simulink model "ControlComparison"  (R2018a)
settings: Solver=VariableStepAuto  StartTime=0  StopTime=4  FixedStep=1e-6
undefined symbols (not defined in the file): alternator, electrical_load, i_f_max, iceToAltRotRatio, n_ice_f, n_ice_i, normalizationFactor, rectifier, t_brake_f, t_brake_i, T_k, T_s
libraries: elec_lib x36, fl_lib x29, nesl_utility x26, neural x25, simulink x6, SimscapeCustomBlocks_lib x2
(part 1 of 3)
settings Model: Creator=gabrielrodrigues  LastModifiedBy=gabriel.rodrigues
settings DataIOCC: ReturnWorkspaceOutputs=on
settings CodeAppCC: StateflowObjectComments=on
settings SimscapeCC: SimscapeNormalizeSystem=off  SimscapeLogType=local  SimscapeLogLimitData=off

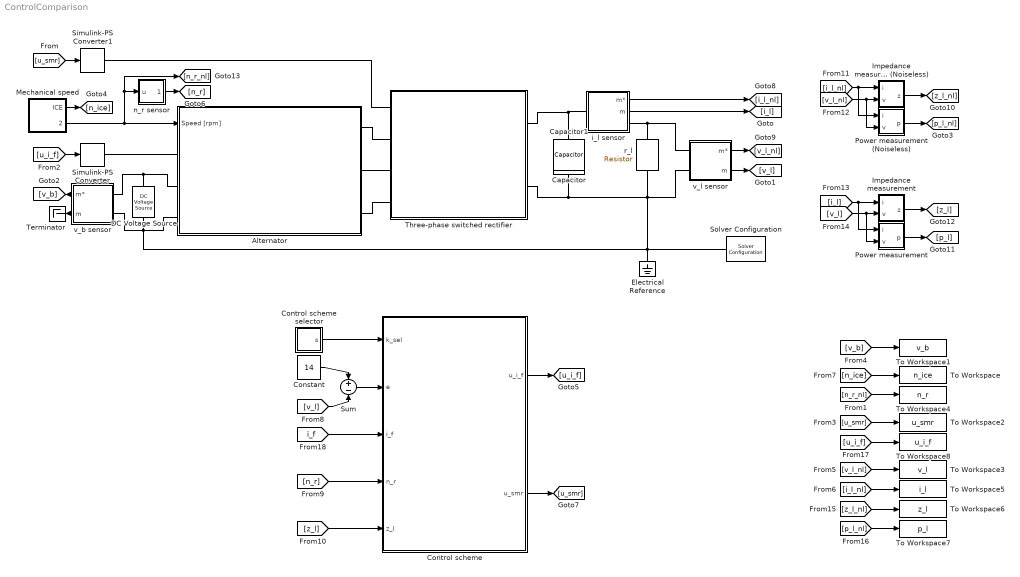
== system ControlComparison ==
  Alternator : Subsystem
  Capacitor : fl_lib/Electrical/Electrical Elements/Capacitor  c=10e-3 F  r=1e-6 Ohm  g=0 1/Ohm  i_specify=off  i_priority=None  i=0 A  i_nominal_specify=off  i_nominal_unit=A  i_nominal_value=1  v_specify=off  v_priority=None  v=0 V  v_nominal_specify=off  v_nominal_unit=V  v_nominal_value=1  vc_specify=off  vc_priority=High  vc=0 V  vc_nominal_specify=off  vc_nominal_unit=V  vc_nominal_value=1
  Capacitor1 : fl_lib/Electrical/Electrical Elements/Capacitor  c=rectifier.filter.c F  r=1e-6 Ohm  g=0 1/Ohm  i_specify=off  i_priority=None  i=0 A  i_nominal_specify=off  i_nominal_unit=A  i_nominal_value=1  v_specify=off  v_priority=None  v=0 V  v_nominal_specify=off  v_nominal_unit=V  v_nominal_value=1  vc_specify=off  vc_priority=High  vc=0 V  vc_nominal_specify=off  vc_nominal_unit=V  vc_nominal_value=1
  Constant : Constant  Value=14
  Control scheme : Subsystem  Variant=on
  Control scheme selector : Subsystem  mask{s_i=0, s_f=1, t_i=t_brake_i, t_f=t_brake_f}
      mask prompts: s_i "Initial value"; s_f "Final value"; t_i "Step start [s]"; t_f "Step end [s]"
  DC Voltage Source : elec_lib/Additional Components/SPICE-Compatible Components/Sources/DC Voltage Source  DC=alternator.rotor.r.value * i_f_max V
      settings: SourceProductName=Simscape Electronics  SourceProductBaseCode=SN
  Electrical Reference : fl_lib/Electrical/Electrical Elements/Electrical Reference
  Impedance measurement : Subsystem
  Impedance measurement (Noiseless) : Subsystem
  Mechanical speed : Subsystem
  Power measurement : Subsystem
  Power measurement (Noiseless) : Subsystem
  Simulink-PS Converter : nesl_utility/Simulink-PS Converter  PhysicalDomain=network_engine_domain  SubClassName=ps_input  LeftPortType=input  RightPortType=output  PseudoPeriodic=off  Frequencies=[]  NoiseDistribution=none  NoiseParameters=[]  Unit=1  AffineConversion=off  FilteringAndDerivatives=provide  SimscapeFilterOrder=1  InputFilterTimeConstant=0.001  UdotUserProvided=0
  Simulink-PS Converter1 : nesl_utility/Simulink-PS Converter  PhysicalDomain=network_engine_domain  SubClassName=ps_input  LeftPortType=input  RightPortType=output  PseudoPeriodic=off  Frequencies=[]  NoiseDistribution=none  NoiseParameters=[]  Unit=1  AffineConversion=off  FilteringAndDerivatives=provide  SimscapeFilterOrder=1  InputFilterTimeConstant=0.001  UdotUserProvided=0
  Solver Configuration : nesl_utility/Solver Configuration  PhysicalDomain=network_engine_domain  SubClassName=solver  LeftPortType=input  RightPortType=generic  Tones=[]  Harmonics=[]  SimulateNoise=off  Profile=off  UseLocalSampling=off  EnableSwitchedLinearOptims=on  FrequencyDomain=off  UseCCode=off  RelTol=0.001  AbsTol=1e-06  MinStep=1e-09  ToWorkspace=off  RevertToSquareIcSolve=off  NumHomotopyIterations=100  PhasorMode=off  PhasorModeNumHarmonics=1  DoDC=on  ResidualTolerance=1e-09  UseLocalSolver=on  LocalSolverChoice=NE_TRAPEZOIDAL_ADVANCER  LocalSolverSampleTime=1e-06  DoFixedCost=on  MaxNonlinIter=20  MaxModeIter=2  LinearAlgebra=Sparse  EquationFormulation=NE_TIME_EF  DelaysMemoryBudget=1024  AutomaticFiltering=on  FilteringTimeConstant=0.001  PartitionStorageMethod=AS_NEEDED  PartitionMemoryBudget=1024
  Sum : Sum  Inputs=+-
  Terminator : Terminator
  Three-phase switched rectifier : Subsystem
  To Workspace : ToWorkspace  VariableName=n_ice  SaveFormat=Timeseries  SampleTime=-1
  To Workspace1 : ToWorkspace  VariableName=v_b  SaveFormat=Timeseries  SampleTime=-1
  To Workspace2 : ToWorkspace  VariableName=u_smr  SaveFormat=Timeseries  SampleTime=-1
  To Workspace3 : ToWorkspace  VariableName=v_l  SaveFormat=Timeseries  SampleTime=-1
  To Workspace4 : ToWorkspace  VariableName=n_r  SaveFormat=Timeseries  SampleTime=-1
  To Workspace5 : ToWorkspace  VariableName=i_l  SaveFormat=Timeseries  SampleTime=-1
  To Workspace6 : ToWorkspace  VariableName=z_l  SaveFormat=Timeseries  SampleTime=-1
  To Workspace7 : ToWorkspace  VariableName=p_l  SaveFormat=Timeseries  SampleTime=-1
  To Workspace8 : ToWorkspace  VariableName=u_i_f  SaveFormat=Timeseries  SampleTime=-1
  i_l sensor : Subsystem
  n_r sensor : Subsystem  mask{T_s=T_s, seed=1515, noise=0.001}
      mask prompts: T_s "Sample time [s]"; noise "Noise percentage"
      mask DialogControl DescGroupVar Prompt: Noisy voltage sensor
  r_l : elec_lib/Passive Devices/Resistor  R=electrical_load.r Ohm  R_tol=5  enable_R_tol=0  tol_distribution=1  nSigma=4  enable_operating_limits=0  operating_limit_action=2  max_working_voltage=100 V  power_rating=1 W  enable_faults=0  fault_action=1  R_faulted=inf Ohm  enable_temporal_fault=0  t_fault=1 s  enable_behavioral_fault=0  max_permissible_current=1 A  t_fail_on_current=1 s  noise_mode=0  sample_time=1e-3 s  repeatability=1  auto_seed=3922919431  user_seed=0  Tdevice=25 degC  alpha=3.93e-3 1/K  Tmeas=25 degC  thermal_mass=100 J/K  power_derating_T1=70 degC  power_derating_T2=155 degC  operating_temperature_range_vec=[-50, 150] degC  temperature_specify=off  temperature_priority=High  temperature=298.15 K  temperature_nominal_specify=off  temperature_nominal_unit=K  temperature_nominal_value=1
  v_b sensor : Subsystem
  v_l sensor : Subsystem
  wires:
  Mechanical speed/2(Alternator) -> [n_r_nl], n_r sensor/1(u), Alternator/1(Speed [rpm])
  [u_i_f] -> Simulink-PS Converter/1
  [u_smr] -> Simulink-PS Converter1/1
  Constant/1 -> Sum/1
  [u_smr] -> To Workspace2/1
  [v_b] -> To Workspace1/1
  [i_l_nl] -> To Workspace5/1
  [v_l_nl] -> To Workspace3/1
  Mechanical speed/1(ICE) -> [n_ice]
  [n_r_nl] -> To Workspace4/1
  [n_ice] -> To Workspace/1
  [v_l] -> Sum/2
  n_r sensor/1(m) -> [n_r]
  v_l sensor/2(m) -> [v_l]
  i_l sensor/2(m) -> [i_l]
  i_l sensor/1(m*) -> [i_l_nl]
  v_l sensor/1(m*) -> [v_l_nl]
  Power measurement (Noiseless)/1(p) -> [p_l_nl]
  Impedance measurement (Noiseless)/1(z) -> [z_l_nl]
  Power measurement/1(p) -> [p_l]
  Impedance measurement/1(z) -> [z_l]
  v_b sensor/1(m*) -> [v_b]
  v_b sensor/2(m) -> Terminator/1
  [i_l_nl] -> Power measurement (Noiseless)/1(i), Impedance measurement (Noiseless)/1(i)
  [v_l_nl] -> Power measurement (Noiseless)/2(v), Impedance measurement (Noiseless)/2(v)
  [v_l] -> Impedance measurement/2(v), Power measurement/2(v)
  [i_l] -> Impedance measurement/1(i), Power measurement/1(i)
  Control scheme/1(u_i_f) -> [u_i_f]
  Control scheme/2(u_smr) -> [u_smr]
  Control scheme selector/1(s) -> Control scheme/1(k_sel)
  [z_l] -> Control scheme/5(z_l)
  [n_r] -> Control scheme/4(n_r)
  Sum/1 -> Control scheme/2(e)
  [p_l_nl] -> To Workspace7/1
  [z_l_nl] -> To Workspace6/1
  [u_i_f] -> To Workspace8/1
  [i_f] -> Control scheme/3(i_f)
  connections:
  Three-phase switched rectifier/LConn3 -- Alternator/RConn2
  Three-phase switched rectifier/LConn4 -- Alternator/RConn3
  Three-phase switched rectifier/LConn2 -- Alternator/RConn1
  Solver Configuration/RConn1 -- Electrical Reference/LConn1 -- v_b sensor/LConn2 -- DC Voltage Source/RConn1 -- Alternator/LConn3 -- r_l/RConn1 -- v_l sensor/LConn2 -- Capacitor/RConn1 -- Three-phase switched rectifier/RConn2
  i_l sensor/RConn1 -- v_l sensor/LConn1 -- r_l/LConn1
  Capacitor/LConn1 -- i_l sensor/LConn1 -- Three-phase switched rectifier/RConn1
  Alternator/LConn2 -- v_b sensor/LConn1 -- DC Voltage Source/LConn1
  Three-phase switched rectifier/LConn1 -- Simulink-PS Converter1/RConn1
  Simulink-PS Converter/RConn1 -- Alternator/LConn1

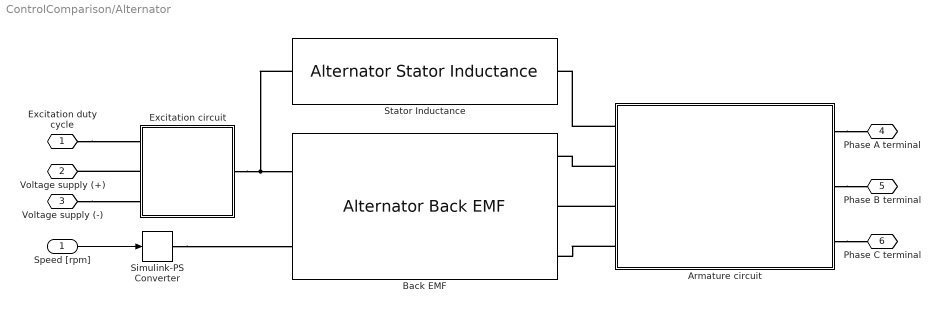
== system ControlComparison/Alternator ==
  Speed [rpm] : Inport
  Armature circuit : Subsystem  Variant=on
  Back EMF : SimscapeCustomBlocks_lib/Alternator/Alternator Back EMF  p=alternator.p  omega_r_specify=off  omega_r_priority=None  omega_r=0 rad/s  omega_r_nominal_specify=off  omega_r_nominal_unit=rad/s  omega_r_nominal_value=1  omega_e_specify=off  omega_e_priority=None  omega_e=0 rad/s  omega_e_nominal_specify=off  omega_e_nominal_unit=rad/s  omega_e_nominal_value=1  k_e_specify=off  k_e_priority=None  k_e=0 s*V/rad/A  k_e_nominal_specify=off  k_e_nominal_unit=s*V/rad/A  k_e_nominal_value=1  e_specify=off  e_priority=None  e=0 rpm  e_nominal_specify=off  e_nominal_unit=rpm  e_nominal_value=1
  Excitation circuit : Subsystem
  Simulink-PS Converter : nesl_utility/Simulink-PS Converter  PhysicalDomain=network_engine_domain  SubClassName=ps_input  LeftPortType=input  RightPortType=output  PseudoPeriodic=off  Frequencies=[]  NoiseDistribution=none  NoiseParameters=[]  Unit=1  AffineConversion=off  FilteringAndDerivatives=provide  SimscapeFilterOrder=1  InputFilterTimeConstant=0.001  UdotUserProvided=0
  Stator Inductance : SimscapeCustomBlocks_lib/Alternator/Alternator Stator Inductance
  Excitation duty cycle : PMIOPort  Side=Left
  Voltage supply (+) : PMIOPort  Port=2  Side=Left
  Voltage supply (-) : PMIOPort  Port=3  Side=Left
  Phase A terminal : PMIOPort  Port=4  Side=Right
  Phase B terminal : PMIOPort  Port=5  Side=Right
  Phase C terminal : PMIOPort  Port=6  Side=Right
  wires:
  Speed [rpm]/1 -> Simulink-PS Converter/1
  connections:
  Armature circuit/RConn1 -- Phase A terminal/RConn1
  Armature circuit/RConn2 -- Phase B terminal/RConn1
  Excitation circuit/LConn2 -- Voltage supply (+)/RConn1
  Voltage supply (-)/RConn1 -- Excitation circuit/LConn3
  Armature circuit/LConn3 -- Back EMF/RConn2
  Armature circuit/LConn2 -- Back EMF/RConn1
  Armature circuit/LConn4 -- Back EMF/RConn3
  Simulink-PS Converter/RConn1 -- Back EMF/LConn2
  Armature circuit/LConn1 -- Stator Inductance/RConn1
  Excitation duty cycle/RConn1 -- Excitation circuit/LConn1
  Excitation circuit/RConn1 -- Stator Inductance/LConn1 -- Back EMF/LConn1
  Armature circuit/RConn3 -- Phase C terminal/RConn1

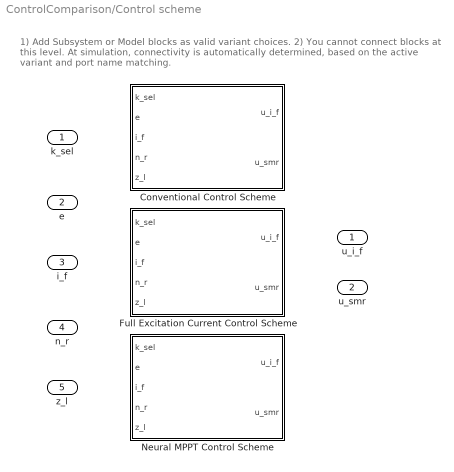
== system ControlComparison/Control scheme ==
  note: 1) Add Subsystem or Model blocks as valid variant choices.
      | 2) You cannot connect blocks at this level. At simulation, connectivity is automatically
      | determined, based on the active variant and port name matching.
  k_sel : Inport
  e : Inport  Port=2
  i_f : Inport  Port=3
  n_r : Inport  Port=4
  z_l : Inport  Port=5
  Conventional Control Scheme : Subsystem  VariantControl=conventionalControlScheme
  Full Excitation Current Control Scheme : Subsystem  VariantControl=fullExcitationCurrentControlScheme
  Neural MPPT Control Scheme : Subsystem  VariantControl=neuralControlScheme
  u_i_f : Outport
  u_smr : Outport  Port=2

== system ControlComparison/Control scheme selector ==
  Step off : Step  Time=t_f  After=s_f - s_i  SampleTime=0
  Step on : Step  Time=t_i  Before=s_i  After=s_f  SampleTime=0
  Sum : Sum  Inputs=+-
  s : Outport
  wires:
  Sum/1 -> s/1
  Step off/1 -> Sum/2
  Step on/1 -> Sum/1

== system ControlComparison/Impedance measurement ==
  i : Inport
  v : Inport  Port=2
  MATLAB Function : MATLAB Function  TreatAsAtomicUnit=on
  z : Outport
  wires:
  i/1 -> MATLAB Function/2(i)
  v/1 -> MATLAB Function/1(v)
  MATLAB Function/1(z) -> z/1

== system ControlComparison/Impedance measurement (Noiseless) ==
  i : Inport
  v : Inport  Port=2
  MATLAB Function : MATLAB Function  TreatAsAtomicUnit=on
  z : Outport
  wires:
  MATLAB Function/1(z) -> z/1
  v/1 -> MATLAB Function/1(v)
  i/1 -> MATLAB Function/2(i)

== system ControlComparison/Mechanical speed ==
  ICE Speed : Subsystem  mask{s_i=n_ice_i, s_f=n_ice_f, t_i=t_brake_i, t_f=t_brake_f}
      mask prompts: s_i "Initial value"; s_f "Final value"; t_i "Ramp start [s]"; t_f "Ramp end [s]"
  ICE to Alternator Rotation Ratio : Constant  Value=iceToAltRotRatio
  Product : Product
  ICE : Outport
  Alternator : Outport  Port=2
  wires:
  ICE Speed/1(s) -> ICE/1, Product/1
  ICE to Alternator Rotation Ratio/1 -> Product/2
  Product/1 -> Alternator/1

== system ControlComparison/Power measurement ==
  i : Inport
  v : Inport  Port=2
  Product : Product
  p : Outport
  wires:
  i/1 -> Product/2
  v/1 -> Product/1
  Product/1 -> p/1

== system ControlComparison/Power measurement (Noiseless) ==
  i : Inport
  v : Inport  Port=2
  Product : Product
  p : Outport
  wires:
  i/1 -> Product/2
  v/1 -> Product/1
  Product/1 -> p/1

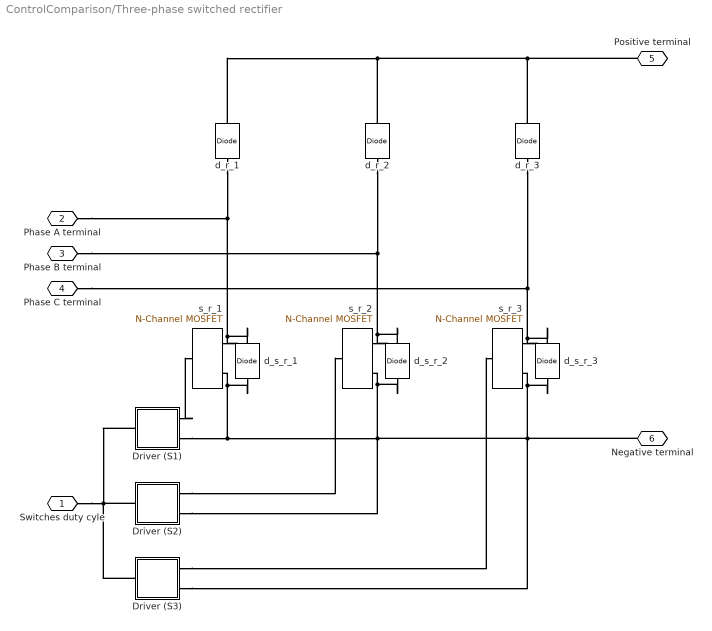
== system ControlComparison/Three-phase switched rectifier ==
  Driver (S1) : Subsystem
  Driver (S2) : Subsystem
  Driver (S3) : Subsystem
  d_r_1 : elec_lib/Semiconductor Devices/Diode  ModelType=1  Vf=rectifier.d.v_on V  Ron=rectifier.d.r_on Ohm  Goff=1e-8 S  Rz=0.3 Ohm  Vz=50 V  C_PWL=5 pF  prmExp=1  I12=[.0137, .545] A  V12=[.6, .7] V  I1=0.0137 A  V1=0.6 V  IS=1e-12 A  ec=1  RS=0.01 Ohm  Tmeas=25 degC  BV=inf V  C_param=1  CJ0=5 pF  VJ=1 V  Mgrad=0.5  Vvec=[.1, 10, 100] V  Cvec=[3.5, 1, .4] pF  FC=0.5  Q_param=1  Irrm=-7.15 A  iF=4 A  didt=-750 A/us  trr=115 ns  TT=50 ns  tau=100 ns  T_param=1  IS_T2=1.25e-7 A  I1_T2=0.245 A  V1_T2=0.5 V  Tmeas2=125 degC  EG_param=1  EG=1.11 eV  XTI_param=1  XTI=3  dBVdT=0 V/K  Tdevice=25 degC  i_capacitor_specify=off  i_capacitor_priority=High  i_capacitor=0 A  i_capacitor_nominal_specify=off  i_capacitor_nominal_unit=A  i_capacitor_nominal_value=1  v_capacitor_specify=off  v_capacitor_priority=None  v_capacitor=0 V  v_capacitor_nominal_specify=off  v_capacitor_nominal_unit=V  v_capacitor_nominal_value=1  Rth=[0, 10] K/W  thermal_mass_parameterization=1  thermal_mass=[0, 1] J/K  thermal_time_constant=[0, 10] s  thermal_mass_initial_temperatures=[25, 25] degC
      settings: SourceProductName=Simscape Electronics  SourceProductBaseCode=SN
  d_r_2 : elec_lib/Semiconductor Devices/Diode  ModelType=1  Vf=rectifier.d.v_on V  Ron=rectifier.d.r_on Ohm  Goff=1e-8 S  Rz=0.3 Ohm  Vz=50 V  C_PWL=5 pF  prmExp=1  I12=[.0137, .545] A  V12=[.6, .7] V  I1=0.0137 A  V1=0.6 V  IS=1e-12 A  ec=1  RS=0.01 Ohm  Tmeas=25 degC  BV=inf V  C_param=1  CJ0=5 pF  VJ=1 V  Mgrad=0.5  Vvec=[.1, 10, 100] V  Cvec=[3.5, 1, .4] pF  FC=0.5  Q_param=1  Irrm=-7.15 A  iF=4 A  didt=-750 A/us  trr=115 ns  TT=50 ns  tau=100 ns  T_param=1  IS_T2=1.25e-7 A  I1_T2=0.245 A  V1_T2=0.5 V  Tmeas2=125 degC  EG_param=1  EG=1.11 eV  XTI_param=1  XTI=3  dBVdT=0 V/K  Tdevice=25 degC  i_capacitor_specify=off  i_capacitor_priority=High  i_capacitor=0 A  i_capacitor_nominal_specify=off  i_capacitor_nominal_unit=A  i_capacitor_nominal_value=1  v_capacitor_specify=off  v_capacitor_priority=None  v_capacitor=0 V  v_capacitor_nominal_specify=off  v_capacitor_nominal_unit=V  v_capacitor_nominal_value=1  Rth=[0, 10] K/W  thermal_mass_parameterization=1  thermal_mass=[0, 1] J/K  thermal_time_constant=[0, 10] s  thermal_mass_initial_temperatures=[25, 25] degC
      settings: SourceProductName=Simscape Electronics  SourceProductBaseCode=SN
  d_r_3 : elec_lib/Semiconductor Devices/Diode  ModelType=1  Vf=rectifier.d.v_on V  Ron=rectifier.d.r_on Ohm  Goff=1e-8 S  Rz=0.3 Ohm  Vz=50 V  C_PWL=5 pF  prmExp=1  I12=[.0137, .545] A  V12=[.6, .7] V  I1=0.0137 A  V1=0.6 V  IS=1e-12 A  ec=1  RS=0.01 Ohm  Tmeas=25 degC  BV=inf V  C_param=1  CJ0=5 pF  VJ=1 V  Mgrad=0.5  Vvec=[.1, 10, 100] V  Cvec=[3.5, 1, .4] pF  FC=0.5  Q_param=1  Irrm=-7.15 A  iF=4 A  didt=-750 A/us  trr=115 ns  TT=50 ns  tau=100 ns  T_param=1  IS_T2=1.25e-7 A  I1_T2=0.245 A  V1_T2=0.5 V  Tmeas2=125 degC  EG_param=1  EG=1.11 eV  XTI_param=1  XTI=3  dBVdT=0 V/K  Tdevice=25 degC  i_capacitor_specify=off  i_capacitor_priority=High  i_capacitor=0 A  i_capacitor_nominal_specify=off  i_capacitor_nominal_unit=A  i_capacitor_nominal_value=1  v_capacitor_specify=off  v_capacitor_priority=None  v_capacitor=0 V  v_capacitor_nominal_specify=off  v_capacitor_nominal_unit=V  v_capacitor_nominal_value=1  Rth=[0, 10] K/W  thermal_mass_parameterization=1  thermal_mass=[0, 1] J/K  thermal_time_constant=[0, 10] s  thermal_mass_initial_temperatures=[25, 25] degC
      settings: SourceProductName=Simscape Electronics  SourceProductBaseCode=SN
  d_s_r_1 : elec_lib/Semiconductor Devices/Diode  ModelType=1  Vf=rectifier.d.v_on V  Ron=rectifier.d.r_on Ohm  Goff=1e-8 S  Rz=0.3 Ohm  Vz=50 V  C_PWL=5 pF  prmExp=1  I12=[.0137, .545] A  V12=[.6, .7] V  I1=0.0137 A  V1=0.6 V  IS=1e-12 A  ec=1  RS=0.01 Ohm  Tmeas=25 degC  BV=inf V  C_param=1  CJ0=5 pF  VJ=1 V  Mgrad=0.5  Vvec=[.1, 10, 100] V  Cvec=[3.5, 1, .4] pF  FC=0.5  Q_param=1  Irrm=-7.15 A  iF=4 A  didt=-750 A/us  trr=115 ns  TT=50 ns  tau=100 ns  T_param=1  IS_T2=1.25e-7 A  I1_T2=0.245 A  V1_T2=0.5 V  Tmeas2=125 degC  EG_param=1  EG=1.11 eV  XTI_param=1  XTI=3  dBVdT=0 V/K  Tdevice=25 degC  i_capacitor_specify=off  i_capacitor_priority=High  i_capacitor=0 A  i_capacitor_nominal_specify=off  i_capacitor_nominal_unit=A  i_capacitor_nominal_value=1  v_capacitor_specify=off  v_capacitor_priority=None  v_capacitor=0 V  v_capacitor_nominal_specify=off  v_capacitor_nominal_unit=V  v_capacitor_nominal_value=1  Rth=[0, 10] K/W  thermal_mass_parameterization=1  thermal_mass=[0, 1] J/K  thermal_time_constant=[0, 10] s  thermal_mass_initial_temperatures=[25, 25] degC
      settings: SourceProductName=Simscape Electronics  SourceProductBaseCode=SN
  d_s_r_2 : elec_lib/Semiconductor Devices/Diode  ModelType=1  Vf=rectifier.d.v_on V  Ron=rectifier.d.r_on Ohm  Goff=1e-8 S  Rz=0.3 Ohm  Vz=50 V  C_PWL=5 pF  prmExp=1  I12=[.0137, .545] A  V12=[.6, .7] V  I1=0.0137 A  V1=0.6 V  IS=1e-12 A  ec=1  RS=0.01 Ohm  Tmeas=25 degC  BV=inf V  C_param=1  CJ0=5 pF  VJ=1 V  Mgrad=0.5  Vvec=[.1, 10, 100] V  Cvec=[3.5, 1, .4] pF  FC=0.5  Q_param=1  Irrm=-7.15 A  iF=4 A  didt=-750 A/us  trr=115 ns  TT=50 ns  tau=100 ns  T_param=1  IS_T2=1.25e-7 A  I1_T2=0.245 A  V1_T2=0.5 V  Tmeas2=125 degC  EG_param=1  EG=1.11 eV  XTI_param=1  XTI=3  dBVdT=0 V/K  Tdevice=25 degC  i_capacitor_specify=off  i_capacitor_priority=High  i_capacitor=0 A  i_capacitor_nominal_specify=off  i_capacitor_nominal_unit=A  i_capacitor_nominal_value=1  v_capacitor_specify=off  v_capacitor_priority=None  v_capacitor=0 V  v_capacitor_nominal_specify=off  v_capacitor_nominal_unit=V  v_capacitor_nominal_value=1  Rth=[0, 10] K/W  thermal_mass_parameterization=1  thermal_mass=[0, 1] J/K  thermal_time_constant=[0, 10] s  thermal_mass_initial_temperatures=[25, 25] degC
      settings: SourceProductName=Simscape Electronics  SourceProductBaseCode=SN
  d_s_r_3 : elec_lib/Semiconductor Devices/Diode  ModelType=1  Vf=rectifier.d.v_on V  Ron=rectifier.d.r_on Ohm  Goff=1e-8 S  Rz=0.3 Ohm  Vz=50 V  C_PWL=5 pF  prmExp=1  I12=[.0137, .545] A  V12=[.6, .7] V  I1=0.0137 A  V1=0.6 V  IS=1e-12 A  ec=1  RS=0.01 Ohm  Tmeas=25 degC  BV=inf V  C_param=1  CJ0=5 pF  VJ=1 V  Mgrad=0.5  Vvec=[.1, 10, 100] V  Cvec=[3.5, 1, .4] pF  FC=0.5  Q_param=1  Irrm=-7.15 A  iF=4 A  didt=-750 A/us  trr=115 ns  TT=50 ns  tau=100 ns  T_param=1  IS_T2=1.25e-7 A  I1_T2=0.245 A  V1_T2=0.5 V  Tmeas2=125 degC  EG_param=1  EG=1.11 eV  XTI_param=1  XTI=3  dBVdT=0 V/K  Tdevice=25 degC  i_capacitor_specify=off  i_capacitor_priority=High  i_capacitor=0 A  i_capacitor_nominal_specify=off  i_capacitor_nominal_unit=A  i_capacitor_nominal_value=1  v_capacitor_specify=off  v_capacitor_priority=None  v_capacitor=0 V  v_capacitor_nominal_specify=off  v_capacitor_nominal_unit=V  v_capacitor_nominal_value=1  Rth=[0, 10] K/W  thermal_mass_parameterization=1  thermal_mass=[0, 1] J/K  thermal_time_constant=[0, 10] s  thermal_mass_initial_temperatures=[25, 25] degC
      settings: SourceProductName=Simscape Electronics  SourceProductBaseCode=SN
  s_r_1 : elec_lib/Semiconductor Devices/N-Channel MOSFET  parameterization=1  prmDatasheet=1  prmEquCoeff=1  Beta=5 A/V^2  Rds=0.025 Ohm  Id=6 A  Vgs=rectifier.s.v_gs_on V  Vth=1.7 V  lam=0 1/V  Tmeas=25 degC  RS=1e-4 Ohm  RD=0.01 Ohm  C_param=1  C_GS=270 pF  C_GD=80 pF  C_DS=0 pF  C_iss=350 pF  C_rss=80 pF  C_oss=0 pF  C_GS_vec=[ 270 300 290 280 295 255 ] pF  C_GD_vec=[ 450 400 300 190 95 55 ] pF  C_DS_vec=[ 450 410 390 230 175 115 ] pF  C_iss_vec=[ 720 700 590 470 390 310 ] pF  C_rss_vec=[ 450 400 300 190 95 55 ] pF  C_oss_vec=[ 900 810 690 420 270 170 ] pF  C_Vds_vec=[ 0.1 0.3 1 3 10 30 ] V  V_GS_for_cap_data=0 V  charge_linearity_param=1  C_OX=200 pF  V_C_OX=-0.5 V  IsDiode=0 A  Vbi=0.6 V  n=1  Cj0Diode=0 pF  TT=50e-9 s  dVth_dT=-6 mV/K  Rds_T2=0.037 Ohm  Tmeas2=125 degC  BEXDatasheet=-1.5  BEXEquCoeff=-1.5  etaisDatasheet=3  etaisEquCoeff=3  TdeviceDatasheet=25 degC  TdeviceEquCoeff=25 degC  Rth=[1, 10] K/W  thermal_mass_parameterization=1  thermal_mass=[1, 1] J/K  thermal_time_constant=[1, 10] s  thermal_mass_initial_temperatures=[ 25 25 ] degC  betaref=18 A/V^2  Vfbref=-1.1 V  gamma=3.5 V^0.50000  phib2ref=1 V  thesatref=0.4 1/V  alpha=0  Vp=5e-2 V  thesrref=0 1/V  m=8  Tref=25 degC  Cox=1500 pF  Cgso=100 pF  Cgdo=14 pF  Rsref=2e-3 Ohm  Rdref=0.17 Ohm  Rgref=8.4 Ohm  Isref=5.2e-13 A  Cj0=480 pF  Tprm=1  etabet=1.3  Stvfb=5e-4 V/K  Stphib=-8.5e-4 V/K  etasat=1.04  etasr=0.65  etar=0.95  etais=3  Tsim=25 degC  T0=[25, 25] degC
      settings: SourceProductName=Simscape Electronics  SourceProductBaseCode=SN  LogSimulationData=on
  s_r_2 : elec_lib/Semiconductor Devices/N-Channel MOSFET  parameterization=1  prmDatasheet=1  prmEquCoeff=1  Beta=5 A/V^2  Rds=0.025 Ohm  Id=6 A  Vgs=rectifier.s.v_gs_on V  Vth=1.7 V  lam=0 1/V  Tmeas=25 degC  RS=1e-4 Ohm  RD=0.01 Ohm  C_param=1  C_GS=270 pF  C_GD=80 pF  C_DS=0 pF  C_iss=350 pF  C_rss=80 pF  C_oss=0 pF  C_GS_vec=[ 270 300 290 280 295 255 ] pF  C_GD_vec=[ 450 400 300 190 95 55 ] pF  C_DS_vec=[ 450 410 390 230 175 115 ] pF  C_iss_vec=[ 720 700 590 470 390 310 ] pF  C_rss_vec=[ 450 400 300 190 95 55 ] pF  C_oss_vec=[ 900 810 690 420 270 170 ] pF  C_Vds_vec=[ 0.1 0.3 1 3 10 30 ] V  V_GS_for_cap_data=0 V  charge_linearity_param=1  C_OX=200 pF  V_C_OX=-0.5 V  IsDiode=0 A  Vbi=0.6 V  n=1  Cj0Diode=0 pF  TT=50e-9 s  dVth_dT=-6 mV/K  Rds_T2=0.037 Ohm  Tmeas2=125 degC  BEXDatasheet=-1.5  BEXEquCoeff=-1.5  etaisDatasheet=3  etaisEquCoeff=3  TdeviceDatasheet=25 degC  TdeviceEquCoeff=25 degC  Rth=[1, 10] K/W  thermal_mass_parameterization=1  thermal_mass=[1, 1] J/K  thermal_time_constant=[1, 10] s  thermal_mass_initial_temperatures=[ 25 25 ] degC  betaref=18 A/V^2  Vfbref=-1.1 V  gamma=3.5 V^0.50000  phib2ref=1 V  thesatref=0.4 1/V  alpha=0  Vp=5e-2 V  thesrref=0 1/V  m=8  Tref=25 degC  Cox=1500 pF  Cgso=100 pF  Cgdo=14 pF  Rsref=2e-3 Ohm  Rdref=0.17 Ohm  Rgref=8.4 Ohm  Isref=5.2e-13 A  Cj0=480 pF  Tprm=1  etabet=1.3  Stvfb=5e-4 V/K  Stphib=-8.5e-4 V/K  etasat=1.04  etasr=0.65  etar=0.95  etais=3  Tsim=25 degC  T0=[25, 25] degC
      settings: SourceProductName=Simscape Electronics  SourceProductBaseCode=SN  LogSimulationData=on
  s_r_3 : elec_lib/Semiconductor Devices/N-Channel MOSFET  parameterization=1  prmDatasheet=1  prmEquCoeff=1  Beta=5 A/V^2  Rds=0.025 Ohm  Id=6 A  Vgs=rectifier.s.v_gs_on V  Vth=1.7 V  lam=0 1/V  Tmeas=25 degC  RS=1e-4 Ohm  RD=0.01 Ohm  C_param=1  C_GS=270 pF  C_GD=80 pF  C_DS=0 pF  C_iss=350 pF  C_rss=80 pF  C_oss=0 pF  C_GS_vec=[ 270 300 290 280 295 255 ] pF  C_GD_vec=[ 450 400 300 190 95 55 ] pF  C_DS_vec=[ 450 410 390 230 175 115 ] pF  C_iss_vec=[ 720 700 590 470 390 310 ] pF  C_rss_vec=[ 450 400 300 190 95 55 ] pF  C_oss_vec=[ 900 810 690 420 270 170 ] pF  C_Vds_vec=[ 0.1 0.3 1 3 10 30 ] V  V_GS_for_cap_data=0 V  charge_linearity_param=1  C_OX=200 pF  V_C_OX=-0.5 V  IsDiode=0 A  Vbi=0.6 V  n=1  Cj0Diode=0 pF  TT=50e-9 s  dVth_dT=-6 mV/K  Rds_T2=0.037 Ohm  Tmeas2=125 degC  BEXDatasheet=-1.5  BEXEquCoeff=-1.5  etaisDatasheet=3  etaisEquCoeff=3  TdeviceDatasheet=25 degC  TdeviceEquCoeff=25 degC  Rth=[1, 10] K/W  thermal_mass_parameterization=1  thermal_mass=[1, 1] J/K  thermal_time_constant=[1, 10] s  thermal_mass_initial_temperatures=[ 25 25 ] degC  betaref=18 A/V^2  Vfbref=-1.1 V  gamma=3.5 V^0.50000  phib2ref=1 V  thesatref=0.4 1/V  alpha=0  Vp=5e-2 V  thesrref=0 1/V  m=8  Tref=25 degC  Cox=1500 pF  Cgso=100 pF  Cgdo=14 pF  Rsref=2e-3 Ohm  Rdref=0.17 Ohm  Rgref=8.4 Ohm  Isref=5.2e-13 A  Cj0=480 pF  Tprm=1  etabet=1.3  Stvfb=5e-4 V/K  Stphib=-8.5e-4 V/K  etasat=1.04  etasr=0.65  etar=0.95  etais=3  Tsim=25 degC  T0=[25, 25] degC
      settings: SourceProductName=Simscape Electronics  SourceProductBaseCode=SN  LogSimulationData=on
  Switches duty cyle : PMIOPort  Side=Left
  Phase A terminal : PMIOPort  Port=2  Side=Left
  Phase B terminal : PMIOPort  Port=3  Side=Left
  Phase C terminal : PMIOPort  Port=4  Side=Left
  Positive terminal : PMIOPort  Port=5  Side=Right
  Negative terminal : PMIOPort  Port=6  Side=Right
  connections:
  Phase B terminal/RConn1 -- d_r_2/LConn1 -- d_s_r_2/RConn1 -- s_r_2/RConn1
  Positive terminal/RConn1 -- d_r_3/RConn1 -- d_r_2/RConn1 -- d_r_1/RConn1
  Phase C terminal/RConn1 -- d_r_3/LConn1 -- d_s_r_3/RConn1 -- s_r_3/RConn1
  Driver (S1)/RConn1 -- s_r_1/LConn1
  Driver (S2)/RConn1 -- s_r_2/LConn1
  Driver (S3)/RConn1 -- s_r_3/LConn1
  Negative terminal/RConn1 -- Driver (S3)/RConn2 -- d_s_r_3/LConn1 -- s_r_3/RConn2 -- Driver (S2)/RConn2 -- Driver (S1)/RConn2 -- d_s_r_1/LConn1 -- s_r_1/RConn2 -- d_s_r_2/LConn1 -- s_r_2/RConn2
  Switches duty cyle/RConn1 -- Driver (S3)/LConn1 -- Driver (S2)/LConn1 -- Driver (S1)/LConn1
  d_s_r_1/RConn1 -- Phase A terminal/RConn1 -- d_r_1/LConn1 -- s_r_1/RConn1

== system ControlComparison/i_l sensor ==
  Current Sensor : Subsystem  mask{T_s=T_k, seed=0, noise=0.05}
      mask prompts: T_s "Sample time [s]"; noise "Noise percentage"
      mask DialogControl DescGroupVar Prompt: Noisy current sensor
  Sample delay : TransferFcn  Denominator=[T_s 1]
  Sample delay1 : TransferFcn  Denominator=[T_s 1]
  + : PMIOPort  Side=Left
  - : PMIOPort  Port=2  Side=Right
  m* : Outport
  m : Outport  Port=2
  wires:
  Sample delay/1 -> m*/1
  Current Sensor/1(m*) -> Sample delay/1
  Current Sensor/2(m) -> Sample delay1/1
  Sample delay1/1 -> m/1
  connections:
  Current Sensor/RConn1 -- -/RConn1
  Current Sensor/LConn1 -- +/RConn1

== system ControlComparison/n_r sensor ==
  u : Inport
  Noise addition : Subsystem  mask{T_s=T_s, seed=seed, noise=noise}
      mask prompts: T_s "Sample time [s]"; noise "Noise percentage"
  m : Outport
  wires:
  Noise addition/1(u + n) -> m/1
  u/1 -> Noise addition/1(u)

== system ControlComparison/v_b sensor ==
  Sample delay : TransferFcn  Denominator=[T_s 1]
  Sample delay1 : TransferFcn  Denominator=[T_s 1]
  Voltage Sensor : Subsystem  mask{T_s=T_k, seed=0, noise=0}
      mask prompts: T_s "Sample time [s]"; noise "Noise percentage"
      mask DialogControl DescGroupVar Prompt: Noisy voltage sensor
  + : PMIOPort  Side=Left
  - : PMIOPort  Port=2  Side=Left
  m* : Outport
  m : Outport  Port=2
  wires:
  Sample delay/1 -> m*/1
  Voltage Sensor/2(m) -> Sample delay1/1
  Sample delay1/1 -> m/1
  Voltage Sensor/1(m*) -> Sample delay/1
  connections:
  -/RConn1 -- Voltage Sensor/LConn2
  +/RConn1 -- Voltage Sensor/LConn1

== system ControlComparison/v_l sensor ==
  Sample delay : TransferFcn  Denominator=[T_s 1]
  Sample delay1 : TransferFcn  Denominator=[T_s 1]
  Voltage Sensor : Subsystem  mask{T_s=T_k, seed=15151, noise=0.05}
      mask prompts: T_s "Sample time [s]"; noise "Noise percentage"
      mask DialogControl DescGroupVar Prompt: Noisy voltage sensor
  + : PMIOPort  Side=Left
  - : PMIOPort  Port=2  Side=Left
  m* : Outport
  m : Outport  Port=2
  wires:
  Sample delay/1 -> m*/1
  Voltage Sensor/2(m) -> Sample delay1/1
  Sample delay1/1 -> m/1
  Voltage Sensor/1(m*) -> Sample delay/1
  connections:
  -/RConn1 -- Voltage Sensor/LConn2
  +/RConn1 -- Voltage Sensor/LConn1

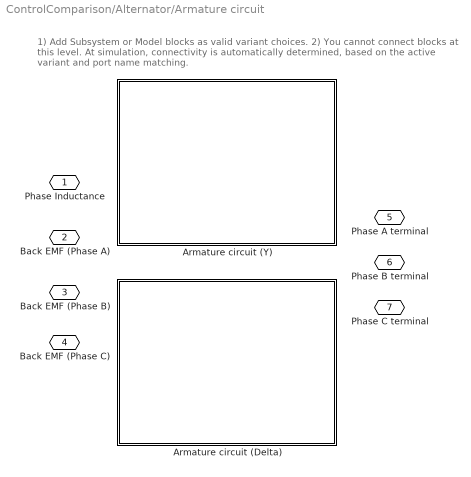
== system ControlComparison/Alternator/Armature circuit ==
  note: 1) Add Subsystem or Model blocks as valid variant choices.
      | 2) You cannot connect blocks at this level. At simulation, connectivity is automatically
      | determined, based on the active variant and port name matching.
  Armature circuit (Delta) : Subsystem  VariantControl=deltaStatorConnection
  Armature circuit (Y) : Subsystem  VariantControl=yStatorConnection
  Phase Inductance : PMIOPort  Side=Left
  Back EMF (Phase A) : PMIOPort  Port=2  Side=Left
  Back EMF (Phase B) : PMIOPort  Port=3  Side=Left
  Back EMF (Phase C) : PMIOPort  Port=4  Side=Left
  Phase A terminal : PMIOPort  Port=5  Side=Right
  Phase B terminal : PMIOPort  Port=6  Side=Right
  Phase C terminal : PMIOPort  Port=7  Side=Right

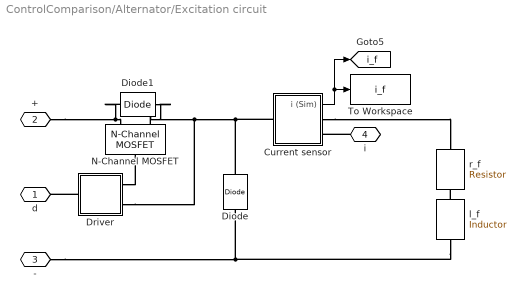
== system ControlComparison/Alternator/Excitation circuit ==
  Current sensor : Subsystem
  Diode : elec_lib/Semiconductor Devices/Diode  ModelType=1  Vf=0.8 V  Ron=10e-3 Ohm  Goff=1e-8 S  Rz=0.3 Ohm  Vz=50 V  C_PWL=5 pF  prmExp=1  I12=[.0137, .545] A  V12=[.6, .7] V  I1=0.0137 A  V1=0.6 V  IS=1e-12 A  ec=1  RS=0.01 Ohm  Tmeas=25 degC  BV=inf V  C_param=1  CJ0=5 pF  VJ=1 V  Mgrad=0.5  Vvec=[.1, 10, 100] V  Cvec=[3.5, 1, .4] pF  FC=0.5  Q_param=1  Irrm=-7.15 A  iF=4 A  didt=-750 A/us  trr=115 ns  TT=50 ns  tau=100 ns  T_param=1  IS_T2=1.25e-7 A  I1_T2=0.245 A  V1_T2=0.5 V  Tmeas2=125 degC  EG_param=1  EG=1.11 eV  XTI_param=1  XTI=3  dBVdT=0 V/K  Tdevice=25 degC  i_capacitor_specify=off  i_capacitor_priority=High  i_capacitor=0 A  i_capacitor_nominal_specify=off  i_capacitor_nominal_unit=A  i_capacitor_nominal_value=1  v_capacitor_specify=off  v_capacitor_priority=None  v_capacitor=0 V  v_capacitor_nominal_specify=off  v_capacitor_nominal_unit=V  v_capacitor_nominal_value=1  Rth=[0, 10] K/W  thermal_mass_parameterization=1  thermal_mass=[0, 1] J/K  thermal_time_constant=[0, 10] s  thermal_mass_initial_temperatures=[25, 25] degC
      settings: SourceProductName=Simscape Electronics  SourceProductBaseCode=SN
  Diode1 : elec_lib/Semiconductor Devices/Diode  ModelType=1  Vf=0.8 V  Ron=10e-3 Ohm  Goff=1e-8 S  Rz=0.3 Ohm  Vz=50 V  C_PWL=5 pF  prmExp=1  I12=[.0137, .545] A  V12=[.6, .7] V  I1=0.0137 A  V1=0.6 V  IS=1e-12 A  ec=1  RS=0.01 Ohm  Tmeas=25 degC  BV=inf V  C_param=1  CJ0=5 pF  VJ=1 V  Mgrad=0.5  Vvec=[.1, 10, 100] V  Cvec=[3.5, 1, .4] pF  FC=0.5  Q_param=1  Irrm=-7.15 A  iF=4 A  didt=-750 A/us  trr=115 ns  TT=50 ns  tau=100 ns  T_param=1  IS_T2=1.25e-7 A  I1_T2=0.245 A  V1_T2=0.5 V  Tmeas2=125 degC  EG_param=1  EG=1.11 eV  XTI_param=1  XTI=3  dBVdT=0 V/K  Tdevice=25 degC  i_capacitor_specify=off  i_capacitor_priority=High  i_capacitor=0 A  i_capacitor_nominal_specify=off  i_capacitor_nominal_unit=A  i_capacitor_nominal_value=1  v_capacitor_specify=off  v_capacitor_priority=None  v_capacitor=0 V  v_capacitor_nominal_specify=off  v_capacitor_nominal_unit=V  v_capacitor_nominal_value=1  Rth=[0, 10] K/W  thermal_mass_parameterization=1  thermal_mass=[0, 1] J/K  thermal_time_constant=[0, 10] s  thermal_mass_initial_temperatures=[25, 25] degC
      settings: SourceProductName=Simscape Electronics  SourceProductBaseCode=SN
  Driver : Subsystem
  N-Channel MOSFET : elec_lib/Semiconductor Devices/N-Channel MOSFET  parameterization=1  prmDatasheet=1  prmEquCoeff=1  Beta=5 A/V^2  Rds=0.025 Ohm  Id=6 A  Vgs=alternator.rotor.s.v_gs_on V  Vth=1.7 V  lam=0 1/V  Tmeas=25 degC  RS=1e-4 Ohm  RD=0.01 Ohm  C_param=1  C_GS=270 pF  C_GD=80 pF  C_DS=0 pF  C_iss=350 pF  C_rss=80 pF  C_oss=0 pF  C_GS_vec=[ 270 300 290 280 295 255 ] pF  C_GD_vec=[ 450 400 300 190 95 55 ] pF  C_DS_vec=[ 450 410 390 230 175 115 ] pF  C_iss_vec=[ 720 700 590 470 390 310 ] pF  C_rss_vec=[ 450 400 300 190 95 55 ] pF  C_oss_vec=[ 900 810 690 420 270 170 ] pF  C_Vds_vec=[ 0.1 0.3 1 3 10 30 ] V  V_GS_for_cap_data=0 V  charge_linearity_param=1  C_OX=200 pF  V_C_OX=-0.5 V  IsDiode=0 A  Vbi=0.6 V  n=1  Cj0Diode=0 pF  TT=50e-9 s  dVth_dT=-6 mV/K  Rds_T2=0.037 Ohm  Tmeas2=125 degC  BEXDatasheet=-1.5  BEXEquCoeff=-1.5  etaisDatasheet=3  etaisEquCoeff=3  TdeviceDatasheet=25 degC  TdeviceEquCoeff=25 degC  Rth=[1, 10] K/W  thermal_mass_parameterization=1  thermal_mass=[1, 1] J/K  thermal_time_constant=[1, 10] s  thermal_mass_initial_temperatures=[ 25 25 ] degC  betaref=18 A/V^2  Vfbref=-1.1 V  gamma=3.5 V^0.50000  phib2ref=1 V  thesatref=0.4 1/V  alpha=0  Vp=5e-2 V  thesrref=0 1/V  m=8  Tref=25 degC  Cox=1500 pF  Cgso=100 pF  Cgdo=14 pF  Rsref=2e-3 Ohm  Rdref=0.17 Ohm  Rgref=8.4 Ohm  Isref=5.2e-13 A  Cj0=480 pF  Tprm=1  etabet=1.3  Stvfb=5e-4 V/K  Stphib=-8.5e-4 V/K  etasat=1.04  etasr=0.65  etar=0.95  etais=3  Tsim=25 degC  T0=[25, 25] degC
      settings: SourceProductName=Simscape Electronics  SourceProductBaseCode=SN
  To Workspace : ToWorkspace  VariableName=i_f  SaveFormat=Timeseries  SampleTime=-1
  l_f : elec_lib/Passive Devices/Inductor  l=alternator.rotor.l.value H  L_tol=20  enable_L_tol=0  tol_distribution=1  nSigma=4  r=0 Ohm  g=1e-9 1/Ohm  enable_operating_limits=0  operating_limit_action=2  max_working_current=1 A  power_rating=1 W  enable_faults=0  fault_action=1  lambdaPercent=50  k_faulted=0.9999  turnsShort=0  openCct=0  groundShort=0  groundShortG=0 1/Ohm  tau_fault=1e-3 s  enable_temporal_fault=0  t_fault=1 s  enable_behavioral_fault=0  max_permissible_voltage=100 V  n_fail_on_voltage=1  max_permissible_current=1 A  t_fail_on_current=1 s  i_L_specify=off  i_L_priority=High  i_L=0 A  i_L_nominal_specify=off  i_L_nominal_unit=A  i_L_nominal_value=1
      settings: SourceProductName=Simscape Electronics  SourceProductBaseCode=SN
  r_f : elec_lib/Passive Devices/Resistor  R=alternator.rotor.r.value Ohm  R_tol=5  enable_R_tol=0  tol_distribution=1  nSigma=4  enable_operating_limits=0  operating_limit_action=2  max_working_voltage=100 V  power_rating=1 W  enable_faults=0  fault_action=1  R_faulted=inf Ohm  enable_temporal_fault=0  t_fault=1 s  enable_behavioral_fault=0  max_permissible_current=1 A  t_fail_on_current=1 s  noise_mode=0  sample_time=1e-3 s  repeatability=1  auto_seed=2791903770  user_seed=0  Tdevice=25 degC  alpha=3.93e-3 1/K  Tmeas=25 degC  thermal_mass=100 J/K  power_derating_T1=70 degC  power_derating_T2=155 degC  operating_temperature_range_vec=[-50.0, 150.0] degC  temperature_specify=off  temperature_priority=High  temperature=298.15 K  temperature_nominal_specify=off  temperature_nominal_unit=K  temperature_nominal_value=1
  d : PMIOPort  Side=Left
  + : PMIOPort  Port=2  Side=Left
  - : PMIOPort  Port=3  Side=Left
  i : PMIOPort  Port=4  Side=Right
  tag scope: i_f=global
  wires:
  Current sensor/1(i (Sim)) -> [i_f], To Workspace/1
  connections:
  l_f/RConn1 -- Diode/LConn1 -- -/RConn1
  +/RConn1 -- Diode1/RConn1 -- N-Channel MOSFET/RConn1
  Current sensor/RConn1 -- r_f/RConn1
  Current sensor/LConn1 -- Diode/RConn1 -- Driver/RConn2 -- Diode1/LConn1 -- N-Channel MOSFET/RConn2
  l_f/LConn1 -- r_f/LConn1
  Driver/RConn1 -- N-Channel MOSFET/LConn1
  i/RConn1 -- Current sensor/RConn2
  Driver/LConn1 -- d/RConn1

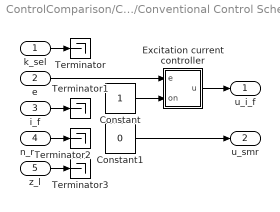
== system ControlComparison/Control scheme/Conventional Control Scheme ==
  k_sel : Inport
  e : Inport  Port=2
  i_f : Inport  Port=3
  n_r : Inport  Port=4
  z_l : Inport  Port=5
  Constant : Constant
  Constant1 : Constant  Value=0
  Excitation current controller : Subsystem
  Terminator{,1..3} (4 alike) : Terminator
  u_i_f : Outport
  u_smr : Outport  Port=2
  wires:
  Constant/1 -> Excitation current controller/2(on)
  e/1 -> Excitation current controller/1(e)
  Excitation current controller/1(u) -> u_i_f/1
  Constant1/1 -> u_smr/1
  k_sel/1 -> Terminator/1
  i_f/1 -> Terminator1/1
  n_r/1 -> Terminator2/1
  z_l/1 -> Terminator3/1

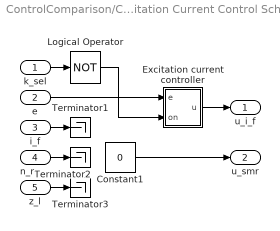
== system ControlComparison/Control scheme/Full Excitation Current Control Scheme ==
  k_sel : Inport
  e : Inport  Port=2
  i_f : Inport  Port=3
  n_r : Inport  Port=4
  z_l : Inport  Port=5
  Constant1 : Constant  Value=0
  Excitation current controller : Subsystem
  Logical Operator : Logic  Operator=NOT  AllPortsSameDT=off  OutDataTypeStr=boolean
  Terminator1 : Terminator
  Terminator2 : Terminator
  Terminator3 : Terminator
  u_i_f : Outport
  u_smr : Outport  Port=2
  wires:
  k_sel/1 -> Logical Operator/1
  e/1 -> Excitation current controller/1(e)
  Excitation current controller/1(u) -> u_i_f/1
  Constant1/1 -> u_smr/1
  Logical Operator/1 -> Excitation current controller/2(on)
  z_l/1 -> Terminator3/1
  i_f/1 -> Terminator1/1
  n_r/1 -> Terminator2/1

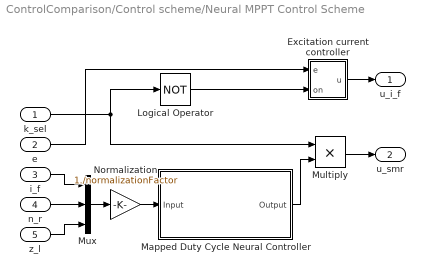
== system ControlComparison/Control scheme/Neural MPPT Control Scheme ==
  k_sel : Inport
  e : Inport  Port=2
  i_f : Inport  Port=3
  n_r : Inport  Port=4
  z_l : Inport  Port=5
  Excitation current controller : Subsystem
  Logical Operator : Logic  Operator=NOT  AllPortsSameDT=off  OutDataTypeStr=boolean
  Mapped Duty Cycle Neural Controller : Subsystem
      mask help: Function Fitting Neural Network
      mask Display: e = 0.06;c1 = [120 150 230]/255;c2 = ([120 150 230]+0)/383;c3 = ([120 150 230]+128)/383;patch([0 1 1 0],[0 0 1 1],c1);patch([0 1 1 1-e 1-e 0+e],[0 0 1 1-e 0+e 0+e],c2);patch([0 0 1 1-e 0+e 0+e],[0 1 1 1-e 1-e 0+e],c3);plot([0 1 1 0 0],[0 0 1 1 0]);fprintf('NNET');port_label('input',1,' Input');port_label('output',1,'Output ');
  Multiply : Product
  Mux : Mux  Inputs=3
  Normalization : Gain  Gain=1./normalizationFactor
  u_i_f : Outport
  u_smr : Outport  Port=2
  wires:
  Logical Operator/1 -> Excitation current controller/2(on)
  n_r/1 -> Mux/2
  i_f/1 -> Mux/1
  Mapped Duty Cycle Neural Controller/1(Output) -> Multiply/2
  k_sel/1 -> Multiply/1, Logical Operator/1
  e/1 -> Excitation current controller/1(e)
  Excitation current controller/1(u) -> u_i_f/1
  Multiply/1 -> u_smr/1
  z_l/1 -> Mux/3
  Mux/1 -> Normalization/1
  Normalization/1 -> Mapped Duty Cycle Neural Controller/1(Input)

== system ControlComparison/Mechanical speed/ICE Speed ==
  Ramp off : simulink/Sources/Ramp  slope=(s_f - s_i)/(t_f - t_i)  start=t_f  InitialOutput=0
  Ramp on : simulink/Sources/Ramp  slope=(s_f - s_i)/(t_f - t_i)  start=t_i  InitialOutput=s_i
  Sum : Sum  Inputs=+-
  s : Outport
  wires:
  Sum/1 -> s/1
  Ramp off/1 -> Sum/2
  Ramp on/1 -> Sum/1

== system ControlComparison/Three-phase switched rectifier/Driver (S1) ==
  Controlled PWM Voltage : elec_lib/Actuators & Drivers/Drivers/Controlled PWM Voltage  F=rectifier.control.pwm.f_s Hz  TD=0 s  pulse_width_offset=0 s  pulse_min=0 s  Vmin=0 V  Vmax=5 V  Vm=5 V  pwm_or_av=1  event_type=2  sample_time=T_s s  u_min=0  u_max=1
      settings: SourceProductName=Simscape Electronics  SourceProductBaseCode=SN
  Electrical Reference : fl_lib/Electrical/Electrical Elements/Electrical Reference
  Gate Driver : elec_lib/Actuators & Drivers/Drivers/Gate Driver  vHigh=rectifier.s.v_gs_on*1.5 V  vLow=0 V  parameterization=1  rHigh=100 Ohm  rLow=10 Ohm  tRise=20 ns  tFall=20 ns  cLoad=10 nF  enable_faults=0  t_fault=1 s  fault_type=1  uHighValue=0.7  uLowValue=0.3  tHigh=50 ns  tLow=100 ns  ZonTime_specify=off  ZonTime_priority=None  ZonTime=0 s  ZoffTime_specify=off  ZoffTime_priority=None  ZoffTime=0 s  uHigh=2.0 V  uLow=0.8 V
      settings: SourceProductName=Simscape Electronics  SourceProductBaseCode=SN
  d : PMIOPort  Side=Left
  v_g : PMIOPort  Port=2  Side=Right
  v_s : PMIOPort  Port=3  Side=Right
  connections:
  Gate Driver/LConn2 -- Controlled PWM Voltage/RConn2 -- Electrical Reference/LConn1
  Controlled PWM Voltage/RConn1 -- Gate Driver/LConn1
  v_g/RConn1 -- Gate Driver/RConn1
  v_s/RConn1 -- Gate Driver/RConn2
  d/RConn1 -- Controlled PWM Voltage/LConn1

== system ControlComparison/Three-phase switched rectifier/Driver (S2) ==
  Controlled PWM Voltage : elec_lib/Actuators & Drivers/Drivers/Controlled PWM Voltage  F=rectifier.control.pwm.f_s Hz  TD=0 s  pulse_width_offset=0 s  pulse_min=0 s  Vmin=0 V  Vmax=5 V  Vm=5 V  pwm_or_av=1  event_type=2  sample_time=T_s s  u_min=0  u_max=1
      settings: SourceProductName=Simscape Electronics  SourceProductBaseCode=SN
  Electrical Reference : fl_lib/Electrical/Electrical Elements/Electrical Reference
  Gate Driver : elec_lib/Actuators & Drivers/Drivers/Gate Driver  vHigh=rectifier.s.v_gs_on*1.5 V  vLow=0 V  parameterization=1  rHigh=100 Ohm  rLow=10 Ohm  tRise=20 ns  tFall=20 ns  cLoad=10 nF  enable_faults=0  t_fault=1 s  fault_type=1  uHighValue=0.7  uLowValue=0.3  tHigh=50 ns  tLow=100 ns  ZonTime_specify=off  ZonTime_priority=None  ZonTime=0 s  ZoffTime_specify=off  ZoffTime_priority=None  ZoffTime=0 s  uHigh=2.0 V  uLow=0.8 V
      settings: SourceProductName=Simscape Electronics  SourceProductBaseCode=SN
  d : PMIOPort  Side=Left
  v_g : PMIOPort  Port=2  Side=Right
  v_s : PMIOPort  Port=3  Side=Right
  connections:
  Gate Driver/LConn2 -- Controlled PWM Voltage/RConn2 -- Electrical Reference/LConn1
  Controlled PWM Voltage/RConn1 -- Gate Driver/LConn1
  v_g/RConn1 -- Gate Driver/RConn1
  v_s/RConn1 -- Gate Driver/RConn2
  d/RConn1 -- Controlled PWM Voltage/LConn1

== system ControlComparison/Three-phase switched rectifier/Driver (S3) ==
  Controlled PWM Voltage : elec_lib/Actuators & Drivers/Drivers/Controlled PWM Voltage  F=rectifier.control.pwm.f_s Hz  TD=0 s  pulse_width_offset=0 s  pulse_min=0 s  Vmin=0 V  Vmax=5 V  Vm=5 V  pwm_or_av=1  event_type=2  sample_time=T_s s  u_min=0  u_max=1
      settings: SourceProductName=Simscape Electronics  SourceProductBaseCode=SN
  Electrical Reference : fl_lib/Electrical/Electrical Elements/Electrical Reference
  Gate Driver : elec_lib/Actuators & Drivers/Drivers/Gate Driver  vHigh=rectifier.s.v_gs_on*1.5 V  vLow=0 V  parameterization=1  rHigh=100 Ohm  rLow=10 Ohm  tRise=20 ns  tFall=20 ns  cLoad=10 nF  enable_faults=0  t_fault=1 s  fault_type=1  uHighValue=0.7  uLowValue=0.3  tHigh=50 ns  tLow=100 ns  ZonTime_specify=off  ZonTime_priority=None  ZonTime=0 s  ZoffTime_specify=off  ZoffTime_priority=None  ZoffTime=0 s  uHigh=2.0 V  uLow=0.8 V
      settings: SourceProductName=Simscape Electronics  SourceProductBaseCode=SN
  d : PMIOPort  Side=Left
  v_g : PMIOPort  Port=2  Side=Right
  v_s : PMIOPort  Port=3  Side=Right
  connections:
  Gate Driver/LConn2 -- Controlled PWM Voltage/RConn2 -- Electrical Reference/LConn1
  Controlled PWM Voltage/RConn1 -- Gate Driver/LConn1
  v_g/RConn1 -- Gate Driver/RConn1
  v_s/RConn1 -- Gate Driver/RConn2
  d/RConn1 -- Controlled PWM Voltage/LConn1

== system ControlComparison/i_l sensor/Current Sensor ==
  Ideal current sensor : Subsystem
  Noise addition : Subsystem  mask{T_s=T_s, seed=seed, noise=noise}
      mask prompts: T_s "Sample time [s]"; noise "Noise percentage"
  + : PMIOPort  Side=Left
  - : PMIOPort  Port=2  Side=Right
  m* : Outport
  m : Outport  Port=2
  wires:
  Ideal current sensor/1(i) -> m*/1, Noise addition/1(u)
  Noise addition/1(u + n) -> m/1
  connections:
  Ideal current sensor/RConn1 -- -/RConn1
  Ideal current sensor/LConn1 -- +/RConn1

== system ControlComparison/n_r sensor/Noise addition ==
  u : Inport
  Band-Limited White Noise : simulink/Sources/Band-Limited White Noise  Cov=[0.1]  Ts=T_s  seed=[seed]
  Gain : Gain  Gain=1/100
  Gain3 : Gain  Gain=noise
  Product2 : Product
  Sum1 : Sum  Inputs=|++
  Zero-Order Hold : ZeroOrderHold  SampleTime=T_s
  u + n : Outport
  wires:
  Gain3/1 -> Product2/1
  Product2/1 -> Sum1/1
  Gain/1 -> Product2/2
  u/1 -> Sum1/2, Gain3/1
  Band-Limited White Noise/1 -> Gain/1
  Sum1/1 -> Zero-Order Hold/1
  Zero-Order Hold/1 -> u + n/1

== system ControlComparison/v_b sensor/Voltage Sensor ==
  Ideal voltage sensor : Subsystem
  Noise addition : Subsystem  mask{T_s=T_s, seed=seed, noise=noise}
      mask prompts: T_s "Sample time [s]"; noise "Noise percentage"
  + : PMIOPort  Side=Left
  - : PMIOPort  Port=2  Side=Left
  m* : Outport
  m : Outport  Port=2
  wires:
  Ideal voltage sensor/1(v) -> m*/1, Noise addition/1(u)
  Noise addition/1(u + n) -> m/1
  connections:
  Ideal voltage sensor/LConn1 -- +/RConn1
  Ideal voltage sensor/RConn1 -- -/RConn1

== system ControlComparison/v_l sensor/Voltage Sensor ==
  Ideal voltage sensor : Subsystem
  Noise addition : Subsystem  mask{T_s=T_s, seed=seed, noise=noise}
      mask prompts: T_s "Sample time [s]"; noise "Noise percentage"
  + : PMIOPort  Side=Left
  - : PMIOPort  Port=2  Side=Left
  m* : Outport
  m : Outport  Port=2
  wires:
  Ideal voltage sensor/1(v) -> m*/1, Noise addition/1(u)
  Noise addition/1(u + n) -> m/1
  connections:
  Ideal voltage sensor/LConn1 -- +/RConn1
  Ideal voltage sensor/RConn1 -- -/RConn1
